simulink model "Lab_5_cart_est"  (R2018a)
settings: Solver=VariableStepAuto  StartTime=0.0  StopTime=10.0  RelTol=1e-3
undefined symbols (not defined in the file): b, M, M1, v0_c
settings Model: Creator=Patrick  LastModifiedBy=Patrick

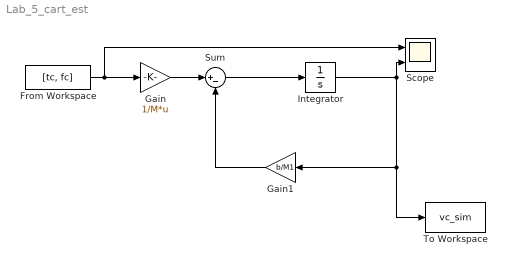
== system Lab_5_cart_est ==
  From Workspace : FromWorkspace  VariableName=[tc, fc]  SampleTime=0
  Gain : Gain  Gain=1/M*u
  Gain1 : Gain  Gain=b/M1
  Integrator : Integrator  InitialCondition=v0_c
  Scope : Scope  NumInputPorts=2
  Sum : Sum  Inputs=|+-
  To Workspace : ToWorkspace  VariableName=vc_sim  SaveFormat=Timeseries  SampleTime=-1
  wires:
  From Workspace/1 -> Scope/1, Gain/1
  Gain/1 -> Sum/1
  Sum/1 -> Integrator/1
  Integrator/1 -> Gain1/1, To Workspace/1, Scope/2
  Gain1/1 -> Sum/2
